simulink model "WT_FFNN_trainbfg_15_15_15_st_2_controller_Oct_6_2023_Nor_0"  (R2021a)
settings: Solver=VariableStepAuto  StartTime=0.0  StopTime=10.0  RelTol=1e-3
libraries: neural x50
(part 2 of 2)

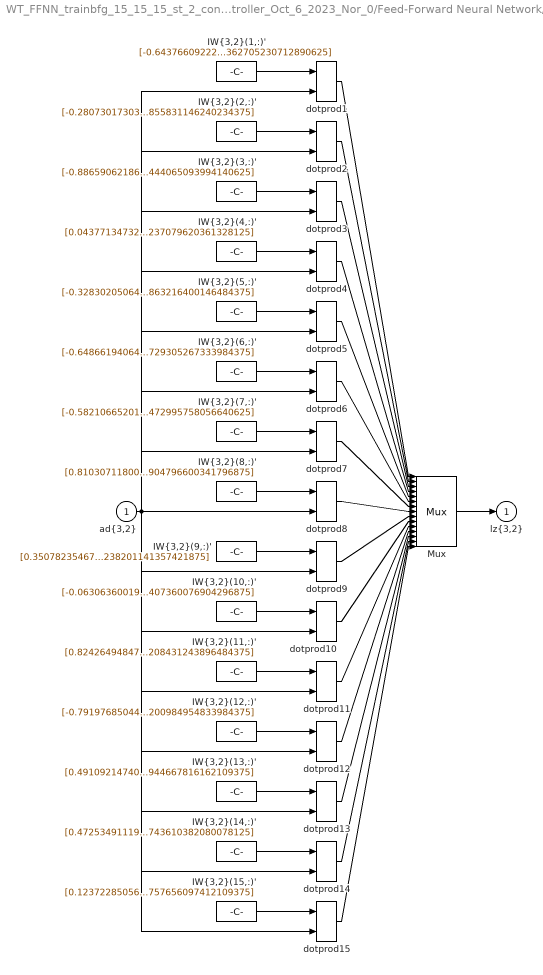
== system WT_FFNN_trainbfg_15_15_15_st_2_controller_Oct_6_2023_Nor_0/Feed-Forward Neural Network/Layer 3/LW{3,2} ==
  "ad{3,2}" : Inport  PortDimensions=15
      mask Display: e = 0.06;c1 = [120 230 180]/255;c2 = ([120 230 180]+0)/(256+128);c3 = ([120 230 180]+128)/(256+128);patch([0 1 1 0],[0 0 1 1],c1);patch([0 1 1 1-e 1-e 0+e],[0 0 1 1-e 0+e 0+e],c2);patch([0 0 1 1-e 0+e 0+e],[0 1 1 1-e 1-e 0+e],c3);plot([0 1 1 0 0],[0 0 1 1 0]);
  "IW{3,2}(1,:)'" : Constant  Value=[-0.643766092226467190329231016221456229686737060546875;-0.63161180496894697711240951321087777614593505859375;-0.0878846663125170124430951545946300029754638671875;0.0675439035340004156893201070488430559635162353515625;0.3850639727730376105085952076478861272335052490234375;-0.897336227775257899708094555535353720188140869140625;0.4800646559755552544856982422061264514923095703125;-0.5886509570704803184781894742627628147602081298828125;-0.7754320756879466980393544872640632092952728271484375;-0.0247924491321527273868241536547429859638214111328125;-0.81529532256159686909313677460886538028717041015625;-0.367142001707418064171406513196416199207305908203125;0.9758694699049907939070180873386561870574951171875;-0.2984465102282147785928145822254009544849395751953125;-0.750254482560374302835271009826101362705230712890625]
      mask Display: e = 0.06;c1 = [120 150 230]/255;c2 = ([120 150 230]+0)/383;c3 = ([120 150 230]+128)/383;patch([0 1 1 0],[0 0 1 1],c1);patch([0 1 1 1-e 1-e 0+e],[0 0 1 1-e 0+e 0+e],c2);patch([0 0 1 1-e 0+e 0+e],[0 1 1 1-e 1-e 0+e],c3);plot([0 1 1 0 0],[0 0 1 1 0]);disp('weights');
  "IW{3,2}(10,:)'" : Constant  Value=[-0.0630636001920052979841102569480426609516143798828125;-0.390097172383417734042865276933298446238040924072265625;0.60375941311085201679276224240311421453952789306640625;0.1709413011814956140366206227554357610642910003662109375;-0.7442232404340096696415685073588974773883819580078125;-1.054724722675212778000286562019027769565582275390625;0.454511728681097848525638482897193171083927154541015625;-0.59364814976334889795595017858431674540042877197265625;0.0259988505286712738573395853336478467099368572235107421875;-0.89646871279220541328669469294254668056964874267578125;-0.6520082622010765494025008592871017754077911376953125;0.740625172065659587161690069478936493396759033203125;0.07284904845598989819865920480879140086472034454345703125;-0.347105338302978072562154920888133347034454345703125;0.5277290128742666563965713066863827407360076904296875]
      mask Display: e = 0.06;c1 = [120 150 230]/255;c2 = ([120 150 230]+0)/383;c3 = ([120 150 230]+128)/383;patch([0 1 1 0],[0 0 1 1],c1);patch([0 1 1 1-e 1-e 0+e],[0 0 1 1-e 0+e 0+e],c2);patch([0 0 1 1-e 0+e 0+e],[0 1 1 1-e 1-e 0+e],c3);plot([0 1 1 0 0],[0 0 1 1 0]);disp('weights');
  "IW{3,2}(11,:)'" : Constant  Value=[0.82426494847924569597807931131683290004730224609375;-0.97808331357209421508258628819021396338939666748046875;0.22787853011803782532496143176103942096233367919921875;0.051869244954289621396537057762543554417788982391357421875;0.0990802140303959077982653980143368244171142578125;0.26797901170358195965803815852268598973751068115234375;0.5720178807069788984307479040580801665782928466796875;-0.53185571195143410694328167664934881031513214111328125;-0.79904957210439853110273134007002227008342742919921875;-0.3683771233222679075680616733734495937824249267578125;-0.8082402700660278327404739684425294399261474609375;0.3766201821637096269768107958952896296977996826171875;-0.6937929329790668564470479395822621881961822509765625;-0.28807496434551971287163496526773087680339813232421875;0.5186494282046554271659033474861644208431243896484375]
      mask Display: e = 0.06;c1 = [120 150 230]/255;c2 = ([120 150 230]+0)/383;c3 = ([120 150 230]+128)/383;patch([0 1 1 0],[0 0 1 1],c1);patch([0 1 1 1-e 1-e 0+e],[0 0 1 1-e 0+e 0+e],c2);patch([0 0 1 1-e 0+e 0+e],[0 1 1 1-e 1-e 0+e],c3);plot([0 1 1 0 0],[0 0 1 1 0]);disp('weights');
  "IW{3,2}(12,:)'" : Constant  Value=[-0.7919768504412429965810815701843239367008209228515625;0.90929301494693504093191904757986776530742645263671875;-1.2307807113800794951430361834354698657989501953125;0.4208026576602830193252202661824412643909454345703125;-0.029541182830081336163630112423561513423919677734375;-0.238439333018778898409806288327672518789768218994140625;-0.469264658498309172873774741674424149096012115478515625;0.09838881490319335842986703255519387312233448028564453125;1.1823087690713973696432503857067786157131195068359375;0.538412375470522786002902648760937154293060302734375;-0.9767276534959286049542015462066046893596649169921875;-0.378896367067337092038314949604682624340057373046875;0.1267465721510132869997988791510579176247119903564453125;-0.292360758968512823852137216817936860024929046630859375;0.481391020687677639866564049953012727200984954833984375]
      mask Display: e = 0.06;c1 = [120 150 230]/255;c2 = ([120 150 230]+0)/383;c3 = ([120 150 230]+128)/383;patch([0 1 1 0],[0 0 1 1],c1);patch([0 1 1 1-e 1-e 0+e],[0 0 1 1-e 0+e 0+e],c2);patch([0 0 1 1-e 0+e 0+e],[0 1 1 1-e 1-e 0+e],c3);plot([0 1 1 0 0],[0 0 1 1 0]);disp('weights');
  "IW{3,2}(13,:)'" : Constant  Value=[0.4910921474034346534409678497468121349811553955078125;-0.454806030865446075939217962513794191181659698486328125;-1.0799356980305778730411248034215532243251800537109375;0.45179230935028968918487635164638049900531768798828125;0.7809513583688765248069785229745320975780487060546875;0.363836622052129909921092121294350363314151763916015625;-0.5940047665978529511932038076338358223438262939453125;-0.81700253732117555927061403053812682628631591796875;-0.777337686148595441437691988539882004261016845703125;0.2490847744972911337324461555908783338963985443115234375;-0.85723783374532924739241934730671346187591552734375;-0.4347099846714741477882171238888986408710479736328125;-0.45490364780995073967773123513325117528438568115234375;0.44249332979861766279583434879896230995655059814453125;0.4873766829746519757549094720161519944667816162109375]
      mask Display: e = 0.06;c1 = [120 150 230]/255;c2 = ([120 150 230]+0)/383;c3 = ([120 150 230]+128)/383;patch([0 1 1 0],[0 0 1 1],c1);patch([0 1 1 1-e 1-e 0+e],[0 0 1 1-e 0+e 0+e],c2);patch([0 0 1 1-e 0+e 0+e],[0 1 1 1-e 1-e 0+e],c3);plot([0 1 1 0 0],[0 0 1 1 0]);disp('weights');
  "IW{3,2}(14,:)'" : Constant  Value=[0.4725349111932770629351807656348682940006256103515625;-0.7762968753872740990118472836911678314208984375;0.1928684866565561206730450294344336725771427154541015625;0.61395379286156537279595113432151265442371368408203125;0.597920557625758686270955877262167632579803466796875;0.61074862905787064004670128269935958087444305419921875;-0.98541176282322873181129807562683708965778350830078125;-0.20052672746393207514614687170251272618770599365234375;-0.05962652359170650395725488124298863112926483154296875;-0.7353695977831105068389661028049886226654052734375;-0.682542723756172531324182273237966001033782958984375;-1.1110063128327245518534027723944745957851409912109375;0.87160267608473318556860931494156830012798309326171875;-0.5761089678544457637343612077529542148113250732421875;-0.7881591665344693797834452198003418743610382080078125]
      mask Display: e = 0.06;c1 = [120 150 230]/255;c2 = ([120 150 230]+0)/383;c3 = ([120 150 230]+128)/383;patch([0 1 1 0],[0 0 1 1],c1);patch([0 1 1 1-e 1-e 0+e],[0 0 1 1-e 0+e 0+e],c2);patch([0 0 1 1-e 0+e 0+e],[0 1 1 1-e 1-e 0+e],c3);plot([0 1 1 0 0],[0 0 1 1 0]);disp('weights');
  "IW{3,2}(15,:)'" : Constant  Value=[0.12372285056327481100879595032893121242523193359375;-0.7535297793022339707391665797331370413303375244140625;1.01284998529049996562889646156691014766693115234375;-0.47101254502392209122518806907464750111103057861328125;0.4686821673919394637408686321577988564968109130859375;-0.193740085798065841959925137416576035320758819580078125;0.933118600820936894280066553619690239429473876953125;-1.0241946624031481594130355006200261414051055908203125;0.2389633859431858631250378266486222855746746063232421875;-0.76070848625679465815352386925951577723026275634765625;-0.237653263205405751445908890673308633267879486083984375;0.21517607246618986049924160397495143115520477294921875;0.50799550266086057614955961980740539729595184326171875;-0.379371279993361454341282978930394165217876434326171875;0.363013506870036584128769163726246915757656097412109375]
      mask Display: e = 0.06;c1 = [120 150 230]/255;c2 = ([120 150 230]+0)/383;c3 = ([120 150 230]+128)/383;patch([0 1 1 0],[0 0 1 1],c1);patch([0 1 1 1-e 1-e 0+e],[0 0 1 1-e 0+e 0+e],c2);patch([0 0 1 1-e 0+e 0+e],[0 1 1 1-e 1-e 0+e],c3);plot([0 1 1 0 0],[0 0 1 1 0]);disp('weights');
  "IW{3,2}(2,:)'" : Constant  Value=[-0.2807301730358393587749787911889143288135528564453125;0.19442270067570976976867314078845083713531494140625;-0.7966612127504897333807321047061122953891754150390625;-0.7816915759150828701962154809734784066677093505859375;0.1133396699280251329611246546846814453601837158203125;-0.854229401802047760838831891305744647979736328125;-0.530346170504191416483763532596640288829803466796875;-0.2234567379043965740237354111741296947002410888671875;0.5688557814878254514923128226655535399913787841796875;0.5379165281177382684774102017399854958057403564453125;-0.9843594128613302185470956828794442117214202880859375;-0.564873381154358700229067835607565939426422119140625;-0.6591359538862333611319854753674007952213287353515625;0.3710714174950744403957969552720896899700164794921875;-0.951131967899252028786349910660646855831146240234375]
      mask Display: e = 0.06;c1 = [120 150 230]/255;c2 = ([120 150 230]+0)/383;c3 = ([120 150 230]+128)/383;patch([0 1 1 0],[0 0 1 1],c1);patch([0 1 1 1-e 1-e 0+e],[0 0 1 1-e 0+e 0+e],c2);patch([0 0 1 1-e 0+e 0+e],[0 1 1 1-e 1-e 0+e],c3);plot([0 1 1 0 0],[0 0 1 1 0]);disp('weights');
  "IW{3,2}(3,:)'" : Constant  Value=[-0.8865906218634176383375233854167163372039794921875;-0.5087226856746489556115875529940240085124969482421875;0.6665547662422302011009378475137054920196533203125;0.4771760059778122897711227778927423059940338134765625;-0.20695841483681487460444259340874850749969482421875;-0.98509372860824451212380381548427976667881011962890625;0.398800633550923377956820559120387770235538482666015625;0.0521827961532089490415131649569957517087459564208984375;-0.5546269515994157739413594754296354949474334716796875;-0.24797594549780910266889577542315237224102020263671875;-0.2343227906718687580944759929479914717376232147216796875;-0.75246930467444428369816478152642957866191864013671875;-0.5304617156856739068615524956840090453624725341796875;-0.46605428111277957814451156082213856279850006103515625;-0.4196294697385456462512820507981814444065093994140625]
      mask Display: e = 0.06;c1 = [120 150 230]/255;c2 = ([120 150 230]+0)/383;c3 = ([120 150 230]+128)/383;patch([0 1 1 0],[0 0 1 1],c1);patch([0 1 1 1-e 1-e 0+e],[0 0 1 1-e 0+e 0+e],c2);patch([0 0 1 1-e 0+e 0+e],[0 1 1 1-e 1-e 0+e],c3);plot([0 1 1 0 0],[0 0 1 1 0]);disp('weights');
  "IW{3,2}(4,:)'" : Constant  Value=[0.0437713473225584959180878286133520305156707763671875;-0.7593750164609780473057298877392895519733428955078125;-0.281448608499250685355264067766256630420684814453125;-0.1798934846500990503148642574160476215183734893798828125;-0.8768186658920706921804821831756271421909332275390625;0.70822561845569576011172330254339613020420074462890625;0.9559435465141794541210629176930524408817291259765625;-0.5502330297056607921746262945816852152347564697265625;0.29247508144850675737558276523486711084842681884765625;-0.45389659936571591369869338450371287763118743896484375;0.41170849539133069772134376762551255524158477783203125;0.84888652171880807362214227396179921925067901611328125;-0.217549552255059619465527021020534448325634002685546875;0.10579682667131480588995628977500018663704395294189453125;-0.3649607741756455414616766574908979237079620361328125]
      mask Display: e = 0.06;c1 = [120 150 230]/255;c2 = ([120 150 230]+0)/383;c3 = ([120 150 230]+128)/383;patch([0 1 1 0],[0 0 1 1],c1);patch([0 1 1 1-e 1-e 0+e],[0 0 1 1-e 0+e 0+e],c2);patch([0 0 1 1-e 0+e 0+e],[0 1 1 1-e 1-e 0+e],c3);plot([0 1 1 0 0],[0 0 1 1 0]);disp('weights');
  "IW{3,2}(5,:)'" : Constant  Value=[-0.3283020506461509224749306667945347726345062255859375;-1.160392655928277338972520738025195896625518798828125;-0.57431761947210813179509614201379008591175079345703125;-0.66366155732263276689764097682200372219085693359375;0.5603510629823471589361361111514270305633544921875;0.5568595499083899280634568640380166471004486083984375;0.7452094051411692898767569204210303723812103271484375;0.09654542970013590963418437240761704742908477783203125;0.749733345695176911505086536635644733905792236328125;-0.925528251189373651897085437667556107044219970703125;0.6545112286603347317992529497132636606693267822265625;0.138648385622836711750238691820413805544376373291015625;-1.2518721770188310227212014069664292037487030029296875;0.7183465107035578167682388084358535706996917724609375;0.30731166956580169280499603701173327863216400146484375]
      mask Display: e = 0.06;c1 = [120 150 230]/255;c2 = ([120 150 230]+0)/383;c3 = ([120 150 230]+128)/383;patch([0 1 1 0],[0 0 1 1],c1);patch([0 1 1 1-e 1-e 0+e],[0 0 1 1-e 0+e 0+e],c2);patch([0 0 1 1-e 0+e 0+e],[0 1 1 1-e 1-e 0+e],c3);plot([0 1 1 0 0],[0 0 1 1 0]);disp('weights');
  "IW{3,2}(6,:)'" : Constant  Value=[-0.6486619406486784367160680631059221923351287841796875;0.79293520498694236575687455115257762372493743896484375;-0.91662855687257416281710220573586411774158477783203125;0.26533309213156319739113087052828632295131683349609375;-0.3248322718959097965552018649759702384471893310546875;0.13292262722521519524576660842285491526126861572265625;-0.8275563483658261443309811511426232755184173583984375;-0.0308438378800735789331266545332255191169679164886474609375;-0.357829990090998195650939806000678800046443939208984375;0.3630397421973954319440736071555875241756439208984375;-0.1432757650358876533314145262920646928250789642333984375;0.052099512431023432823540275649065733887255191802978515625;0.46371881759015709523197301678010262548923492431640625;0.0468194515362923835422037655007443390786647796630859375;0.91387184814136812605056547909043729305267333984375]
      mask Display: e = 0.06;c1 = [120 150 230]/255;c2 = ([120 150 230]+0)/383;c3 = ([120 150 230]+128)/383;patch([0 1 1 0],[0 0 1 1],c1);patch([0 1 1 1-e 1-e 0+e],[0 0 1 1-e 0+e 0+e],c2);patch([0 0 1 1-e 0+e 0+e],[0 1 1 1-e 1-e 0+e],c3);plot([0 1 1 0 0],[0 0 1 1 0]);disp('weights');
  "IW{3,2}(7,:)'" : Constant  Value=[-0.582106652013729242156614418490789830684661865234375;-0.8570943744259109653427231023670174181461334228515625;-0.40351205622447228194005219847895205020904541015625;-0.979326763313207226957501916331239044666290283203125;0.215731814525891518741218533250503242015838623046875;-0.735834088572874467359952177503146231174468994140625;-0.2671267673616022353400012434576638042926788330078125;-0.6963089497674668226778749158256687223911285400390625;0.3895043892358802661846084447461180388927459716796875;-0.14087108149629390396739836432971060276031494140625;-0.782364123453909154903840317274443805217742919921875;-0.631132664484693517437108312151394784450531005859375;-0.19522333460767615775921512977220118045806884765625;-0.3293773385895077954188536750734783709049224853515625;0.8714617455697608594533676296123303472995758056640625]
      mask Display: e = 0.06;c1 = [120 150 230]/255;c2 = ([120 150 230]+0)/383;c3 = ([120 150 230]+128)/383;patch([0 1 1 0],[0 0 1 1],c1);patch([0 1 1 1-e 1-e 0+e],[0 0 1 1-e 0+e 0+e],c2);patch([0 0 1 1-e 0+e 0+e],[0 1 1 1-e 1-e 0+e],c3);plot([0 1 1 0 0],[0 0 1 1 0]);disp('weights');
  "IW{3,2}(8,:)'" : Constant  Value=[0.8103071180089280733938039702479727566242218017578125;-0.87124174673683951741764985854388214647769927978515625;-0.84337858170896951026662691219826228916645050048828125;-1.037872504291950548349632299505174160003662109375;0.4825080990044359197099765879102051258087158203125;0.60300279768864284424267907525063492357730865478515625;-0.303326199032858401238854639814235270023345947265625;0.563864440430446478558224043808877468109130859375;0.75590208909314016150204906807630322873592376708984375;-0.0969098367395359872045190741118858568370342254638671875;0.42807111167921518823931137376348488032817840576171875;-0.63791900559639136414347149184322915971279144287109375;0.613320543020368091902128071524202823638916015625;-0.1521582371998323746087322660969221033155918121337890625;-0.084227332291266332475743183749727904796600341796875]
      mask Display: e = 0.06;c1 = [120 150 230]/255;c2 = ([120 150 230]+0)/383;c3 = ([120 150 230]+128)/383;patch([0 1 1 0],[0 0 1 1],c1);patch([0 1 1 1-e 1-e 0+e],[0 0 1 1-e 0+e 0+e],c2);patch([0 0 1 1-e 0+e 0+e],[0 1 1 1-e 1-e 0+e],c3);plot([0 1 1 0 0],[0 0 1 1 0]);disp('weights');
  "IW{3,2}(9,:)'" : Constant  Value=[0.35078235467249374579523646389134228229522705078125;-0.892491215582572383624437861726619303226470947265625;0.010856284915405911561947505106218159198760986328125;0.3358322431472473557079183592577464878559112548828125;-0.7903735160530007686219278184580616652965545654296875;-0.7792930387153027549373973670299164950847625732421875;0.3700569453232185335167514494969509541988372802734375;-0.7987873552751569850016721829888410866260528564453125;-0.1347153477057989601206600127625279128551483154296875;0.2197143385804321003007544277352280914783477783203125;-0.7470002693413941852185189418378286063671112060546875;-0.8453063837746463971001276149763725697994232177734375;-0.195632029555030673151350129046477377414703369140625;-0.0948149168613519055526239753817208111286163330078125;-0.5190432063358307868128349582548253238201141357421875]
      mask Display: e = 0.06;c1 = [120 150 230]/255;c2 = ([120 150 230]+0)/383;c3 = ([120 150 230]+128)/383;patch([0 1 1 0],[0 0 1 1],c1);patch([0 1 1 1-e 1-e 0+e],[0 0 1 1-e 0+e 0+e],c2);patch([0 0 1 1-e 0+e 0+e],[0 1 1 1-e 1-e 0+e],c3);plot([0 1 1 0 0],[0 0 1 1 0]);disp('weights');
  Mux : Mux  Inputs=15
      mask Display: e = 0.06;c1 = [120 150 230]/255;c2 = ([120 150 230]+0)/383;c3 = ([120 150 230]+128)/383;patch([0 1 1 0],[0 0 1 1],c1);patch([0 1 1 1-e 1-e 0+e],[0 0 1 1-e 0+e 0+e],c2);patch([0 0 1 1-e 0+e 0+e],[0 1 1 1-e 1-e 0+e],c3);plot([0 1 1 0 0],[0 0 1 1 0]);disp('Mux');
  dotprod{1..15} (15 alike) : neural/Weight Functions/dotprod
  "lz{3,2}" : Outport
      mask Display: e = 0.06;c1 = [120 230 180]/255;c2 = ([120 230 180]+0)/(256+128);c3 = ([120 230 180]+128)/(256+128);patch([0 1 1 0],[0 0 1 1],c1);patch([0 1 1 1-e 1-e 0+e],[0 0 1 1-e 0+e 0+e],c2);patch([0 0 1 1-e 0+e 0+e],[0 1 1 1-e 1-e 0+e],c3);plot([0 1 1 0 0],[0 0 1 1 0]);
  wires:
  "IW{3,2}(1,:)'"/1 -> dotprod1/1
  "ad{3,2}"/1 -> dotprod1/2, dotprod2/2, dotprod3/2, dotprod4/2, dotprod5/2, dotprod6/2, dotprod7/2, dotprod8/2, dotprod9/2, dotprod10/2, dotprod11/2, dotprod12/2, dotprod13/2, dotprod14/2, dotprod15/2
  dotprod1/1 -> Mux/1
  "IW{3,2}(2,:)'"/1 -> dotprod2/1
  dotprod2/1 -> Mux/2
  "IW{3,2}(3,:)'"/1 -> dotprod3/1
  dotprod3/1 -> Mux/3
  "IW{3,2}(4,:)'"/1 -> dotprod4/1
  dotprod4/1 -> Mux/4
  "IW{3,2}(5,:)'"/1 -> dotprod5/1
  dotprod5/1 -> Mux/5
  "IW{3,2}(6,:)'"/1 -> dotprod6/1
  dotprod6/1 -> Mux/6
  "IW{3,2}(7,:)'"/1 -> dotprod7/1
  dotprod7/1 -> Mux/7
  "IW{3,2}(8,:)'"/1 -> dotprod8/1
  dotprod8/1 -> Mux/8
  "IW{3,2}(9,:)'"/1 -> dotprod9/1
  dotprod9/1 -> Mux/9
  "IW{3,2}(10,:)'"/1 -> dotprod10/1
  dotprod10/1 -> Mux/10
  "IW{3,2}(11,:)'"/1 -> dotprod11/1
  dotprod11/1 -> Mux/11
  "IW{3,2}(12,:)'"/1 -> dotprod12/1
  dotprod12/1 -> Mux/12
  "IW{3,2}(13,:)'"/1 -> dotprod13/1
  dotprod13/1 -> Mux/13
  "IW{3,2}(14,:)'"/1 -> dotprod14/1
  dotprod14/1 -> Mux/14
  "IW{3,2}(15,:)'"/1 -> dotprod15/1
  dotprod15/1 -> Mux/15
  Mux/1 -> "lz{3,2}"/1

== system WT_FFNN_trainbfg_15_15_15_st_2_controller_Oct_6_2023_Nor_0/Feed-Forward Neural Network/Layer 4/Delays 1 ==
  "p{4}" : Inport  PortDimensions=15
      mask Display: e = 0.06;c1 = [120 230 180]/255;c2 = ([120 230 180]+0)/(256+128);c3 = ([120 230 180]+128)/(256+128);patch([0 1 1 0],[0 0 1 1],c1);patch([0 1 1 1-e 1-e 0+e],[0 0 1 1-e 0+e 0+e],c2);patch([0 0 1 1-e 0+e 0+e],[0 1 1 1-e 1-e 0+e],c3);plot([0 1 1 0 0],[0 0 1 1 0]);
  mux : Mux  Inputs=1
      mask Display: e = 0.06;c1 = [120 150 230]/255;c2 = ([120 150 230]+0)/383;c3 = ([120 150 230]+128)/383;patch([0 1 1 0],[0 0 1 1],c1);patch([0 1 1 1-e 1-e 0+e],[0 0 1 1-e 0+e 0+e],c2);patch([0 0 1 1-e 0+e 0+e],[0 1 1 1-e 1-e 0+e],c3);plot([0 1 1 0 0],[0 0 1 1 0]);disp('Mux')
  "pd{4,3}" : Outport
      mask Display: e = 0.06;c1 = [120 230 180]/255;c2 = ([120 230 180]+0)/(256+128);c3 = ([120 230 180]+128)/(256+128);patch([0 1 1 0],[0 0 1 1],c1);patch([0 1 1 1-e 1-e 0+e],[0 0 1 1-e 0+e 0+e],c2);patch([0 0 1 1-e 0+e 0+e],[0 1 1 1-e 1-e 0+e],c3);plot([0 1 1 0 0],[0 0 1 1 0]);
  wires:
  "p{4}"/1 -> mux/1
  mux/1 -> "pd{4,3}"/1

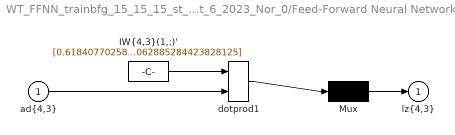
== system WT_FFNN_trainbfg_15_15_15_st_2_controller_Oct_6_2023_Nor_0/Feed-Forward Neural Network/Layer 4/LW{4,3} ==
  "ad{4,3}" : Inport  PortDimensions=15
      mask Display: e = 0.06;c1 = [120 230 180]/255;c2 = ([120 230 180]+0)/(256+128);c3 = ([120 230 180]+128)/(256+128);patch([0 1 1 0],[0 0 1 1],c1);patch([0 1 1 1-e 1-e 0+e],[0 0 1 1-e 0+e 0+e],c2);patch([0 0 1 1-e 0+e 0+e],[0 1 1 1-e 1-e 0+e],c3);plot([0 1 1 0 0],[0 0 1 1 0]);
  "IW{4,3}(1,:)'" : Constant  Value=[0.61840770258758670507859278586693108081817626953125;0.4972377435523942512674011595663614571094512939453125;-0.7184060469143316307594204772613011300563812255859375;-0.19428134296874188802206617765477858483791351318359375;-0.591520851510869416500781881040893495082855224609375;0.50127743350030462554656196516589261591434478759765625;-0.20223849523360204472055556834675371646881103515625;-1.1100369880385028142910641690832562744617462158203125;-0.63852447949041124530822344240732491016387939453125;-0.5392130409800548473953085704124532639980316162109375;-0.96032080944593223303940021651214919984340667724609375;1.636442862890155058863683734671212732791900634765625;0.6544112569637141607614694294170476496219635009765625;1.2622080761251088798502451027161441743373870849609375;-1.0621699197328482444646624571760185062885284423828125]
      mask Display: e = 0.06;c1 = [120 150 230]/255;c2 = ([120 150 230]+0)/383;c3 = ([120 150 230]+128)/383;patch([0 1 1 0],[0 0 1 1],c1);patch([0 1 1 1-e 1-e 0+e],[0 0 1 1-e 0+e 0+e],c2);patch([0 0 1 1-e 0+e 0+e],[0 1 1 1-e 1-e 0+e],c3);plot([0 1 1 0 0],[0 0 1 1 0]);disp('weights');
  Mux : Mux  Inputs=1
      mask Display: e = 0.06;c1 = [120 150 230]/255;c2 = ([120 150 230]+0)/383;c3 = ([120 150 230]+128)/383;patch([0 1 1 0],[0 0 1 1],c1);patch([0 1 1 1-e 1-e 0+e],[0 0 1 1-e 0+e 0+e],c2);patch([0 0 1 1-e 0+e 0+e],[0 1 1 1-e 1-e 0+e],c3);plot([0 1 1 0 0],[0 0 1 1 0]);disp('Mux');
  dotprod1 : neural/Weight Functions/dotprod
  "lz{4,3}" : Outport
      mask Display: e = 0.06;c1 = [120 230 180]/255;c2 = ([120 230 180]+0)/(256+128);c3 = ([120 230 180]+128)/(256+128);patch([0 1 1 0],[0 0 1 1],c1);patch([0 1 1 1-e 1-e 0+e],[0 0 1 1-e 0+e 0+e],c2);patch([0 0 1 1-e 0+e 0+e],[0 1 1 1-e 1-e 0+e],c3);plot([0 1 1 0 0],[0 0 1 1 0]);
  wires:
  "IW{4,3}(1,:)'"/1 -> dotprod1/1
  "ad{4,3}"/1 -> dotprod1/2
  dotprod1/1 -> Mux/1
  Mux/1 -> "lz{4,3}"/1
